simulink model "pod_trav"  (R2022b)
settings: Solver=VariableStepAuto  StartTime=0.0  StopTime=10.0  RelTol=1e-3
undefined symbols (not defined in the file or in its folder): fix_constt, JLrtg, JLrtt, JMrtg, JMrtt, Kktt, Kvtt
settings Model: Creator=ohadformanair  LastModifiedBy=ohadformanair

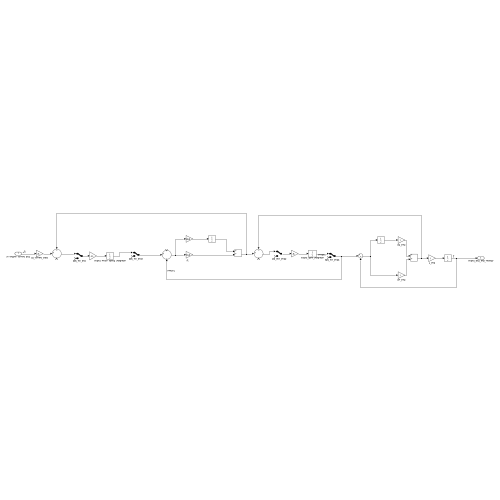
[thumbnail: Simulink's stored preview of the top-level diagram]
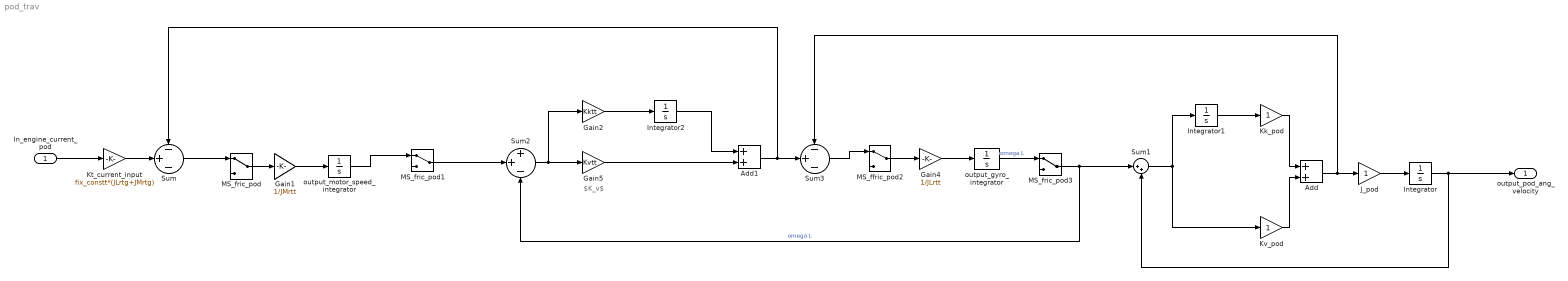
== system pod_trav ==
  note: $K_v$
  In_engine_current_pod : Inport
  Add : Sum
  Add1 : Sum
  Gain1 : Gain  Gain=1/JMrtt
  Gain2 : Gain  Gain=Kktt
  Gain4 : Gain  Gain=1/JLrtt
  Gain5 : Gain  Gain=Kvtt
  Integrator : Integrator
  Integrator1 : Integrator
  Integrator2 : Integrator
  J_pod : Gain
  Kk_pod : Gain
  Kt_current_input : Gain  Gain=fix_constt*(JLrtg+JMrtg)
  Kv_pod : Gain
  MS_ffric_pod2 : ManualSwitch
  MS_fric_pod : ManualSwitch
  MS_fric_pod1 : ManualSwitch
  MS_fric_pod3 : ManualSwitch
  Sum : Sum  Inputs=-+-
  Sum1 : Sum  Inputs=|++
  Sum2 : Sum  Inputs=++-
  Sum3 : Sum  Inputs=-+-
  output_gyro_integrator : Integrator
  output_motor_speed_integrator : Integrator
  output_pod_ang_velocity : Outport
  wires:
  Kv_pod/1 -> Add/2
  J_pod/1 -> Integrator/1
  Kk_pod/1 -> Add/1
  Integrator1/1 -> Kk_pod/1
  Sum1/1 -> Kv_pod/1, Integrator1/1
  Add/1 -> Sum3/1, J_pod/1
  Integrator/1 -> output_pod_ang_velocity/1, Sum1/2
  Gain2/1 -> Integrator2/1
  Gain1/1 -> output_motor_speed_integrator/1
  Integrator2/1 -> Add1/1
  Gain4/1 -> output_gyro_integrator/1
  Gain5/1 -> Add1/2
  MS_ffric_pod2/1 -> Gain4/1
  MS_fric_pod3/1 -> Sum1/1, Sum2/3  "omega L"
  Sum3/1 -> MS_ffric_pod2/1
  MS_fric_pod1/1 -> Sum2/2
  Add1/1 -> Sum3/2, Sum/1
  MS_fric_pod/1 -> Gain1/1
  Sum/1 -> MS_fric_pod/1
  Kt_current_input/1 -> Sum/2
  output_motor_speed_integrator/1 -> MS_fric_pod1/1
  output_gyro_integrator/1 -> MS_fric_pod3/1  "omega L"
  In_engine_current_pod/1 -> Kt_current_input/1
  Sum2/1 -> Gain2/1, Gain5/1
